simulink model "SchemaBlocs"  (R2021b)
settings: Solver=VariableStepAuto  StartTime=0.0  StopTime=10.0  RelTol=1e-3
libraries: slctrlblks x1, simulink x1
settings Model: Creator=xavier.pessoles2  LastModifiedBy=xavier.pessoles2

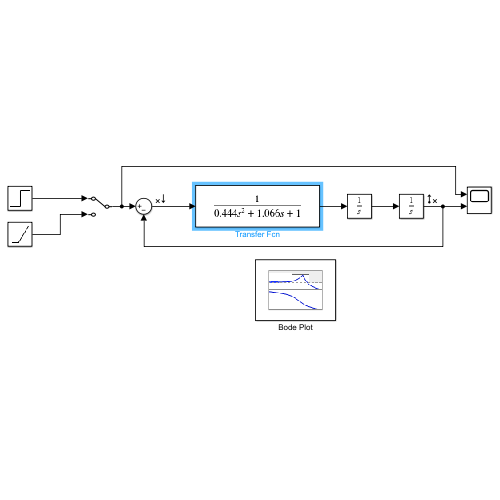
[thumbnail: Simulink's stored preview of the top-level diagram]
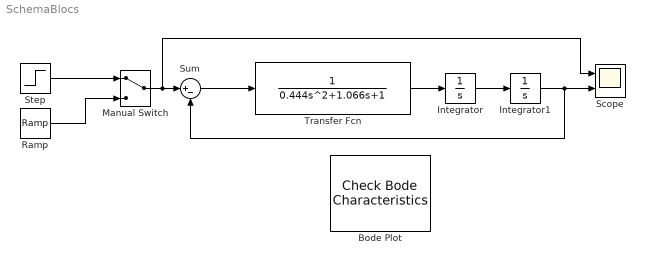
== system SchemaBlocs ==
  Bode Plot : slctrlblks/Model Verification/Check Bode  Characteristics  InstantiateOnLoad=on  SaveOperatingPoints=off  LinearizationIOs={'/Sum', 1, 'in', 'on', '';'/Integrator1', 1, 'out', 'on', ''}  LinearizeAt=SnapshotTimes  SnapshotTimes=[0]  TriggerType=rising  SampleTime=auto  RateConversionMethod=zoh  PreWarpFreq=10  UseExactDelayModel=off  UseFullBlockNameLabels=off  UseBusSignalLabels=off  enabled=on  stopWhenAssertionFail=off  export=off  ViewDlgPos=[842 42 838 426]  OpenViewOnLoad=on  LaunchViewOnOpen=on  FrequencyUnits=rad/s  MagnitudeUnits=dB  PhaseUnits=deg  TimeUnits=seconds  EnableUpperBound=off  UpperBoundFrequencies=[]  UpperBoundMagnitudes=[]  EnableLowerBound=off  LowerBoundFrequencies=[]  LowerBoundMagnitudes=[]
  Integrator : Integrator
  Integrator1 : Integrator
  Manual Switch : ManualSwitch
  Ramp : simulink/Sources/Ramp  slope=1  start=0  InitialOutput=0
  Scope : Scope  NumInputPorts=2
  Step : Step  Time=0  After=300  SampleTime=0
  Sum : Sum  Inputs=|+-
  Transfer Fcn : TransferFcn  Denominator=[0.444 1.066 1]
  wires:
  Transfer Fcn/1 -> Integrator/1
  Integrator/1 -> Integrator1/1
  Sum/1 -> Transfer Fcn/1
  Integrator1/1 -> Scope/2, Sum/2
  Manual Switch/1 -> Scope/1, Sum/1
  Step/1 -> Manual Switch/1
  Ramp/1 -> Manual Switch/2
